simulink model "segway_control"  (R2019b)
settings: Solver=ode45  StartTime=0.0  StopTime=5  MaxStep=0.01  RelTol=1e-3
values from neighbouring files (symbols this model uses):
  A_pitch = [0    1     0     0 ... (first row only)    [vehiculo_autobalanceado_ss.m]
  A_yaw = [0  1 ... (first row only)    [vehiculo_autobalanceado_ss.m]
  B_pitch = [0 ... (first row only)    [vehiculo_autobalanceado_ss.m]
  B_yaw = [0 ... (first row only)    [vehiculo_autobalanceado_ss.m]
  C_pitch = [1 0 0 0 ... (first row only)    [vehiculo_autobalanceado_ss.m]
  C_yaw = [1 0]    [vehiculo_autobalanceado_ss.m]
  D_pitch = zeros(2, 1)    [vehiculo_autobalanceado_ss.m]
  D_yaw = 0    [vehiculo_autobalanceado_ss.m]
libraries: simulink x2
settings Model: Creator=crist  LastModifiedBy=crist

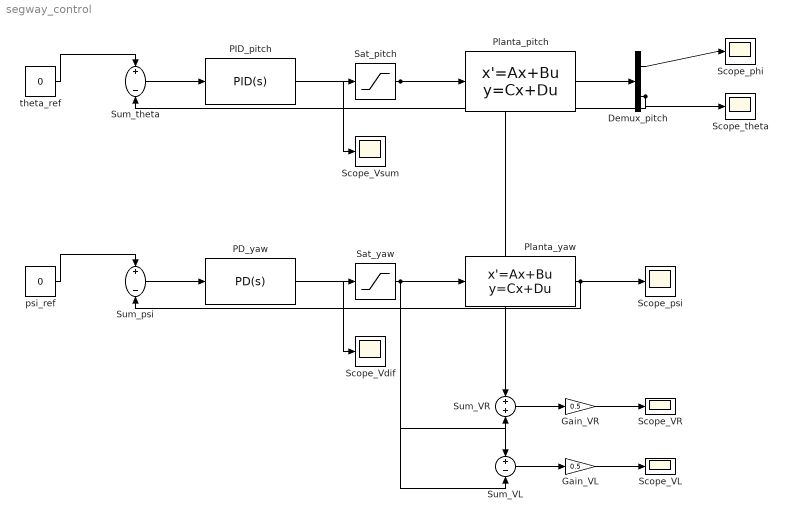
== system segway_control ==
  Demux_pitch : Demux  Outputs=2
  Gain_VL : Gain  Gain=0.5
  Gain_VR : Gain  Gain=0.5
  PD_yaw : simulink/Continuous/PID Controller  Controller=PD  Form=Parallel  TimeDomain=Continuous-time  SampleTime=-1  IntegratorMethod=Forward Euler  FilterMethod=Forward Euler  ControllerParametersSource=internal  P=2  I=1  D=0.3  UseFilter=on  N=100  TunerSelectOption=Transfer Function Based (PID Tuner App)  InitialConditionSource=internal  InitialConditionForIntegrator=0  InitialConditionForFilter=0  DifferentiatorICPrevScaledInput=0  ExternalReset=none  TrackingMode=off  Kt=1  LimitOutput=off  UpperSaturationLimit=inf  LowerSaturationLimit=-inf  LinearizeAsGain=on  AntiWindupMode=none  Kb=1  POutMin=[]  POutMax=[]  IOutMin=[]  IOutMax=[]  DOutMin=[]  DOutMax=[]  NOutMin=[]  NOutMax=[]  SumOutMin=[]  SumOutMax=[]  SaturationOutMin=[]  SaturationOutMax=[]  PParamMin=[]  PParamMax=[]  IParamMin=[]  IParamMax=[]  DParamMin=[]  DParamMax=[]  NParamMin=[]  NParamMax=[]  KbParamMin=[]  KbParamMax=[]  KtParamMin=[]  KtParamMax=[]  KbOutMin=[]  KbOutMax=[]  KtOutMin=[]  KtOutMax=[]  IntegratorOutMin=[]  IntegratorOutMax=[]  FilterOutMin=[]  FilterOutMax=[]  SumI1OutMin=[]  SumI1OutMax=[]  SumI2OutMin=[]  SumI2OutMax=[]  SumI3OutMin=[]  SumI3OutMax=[]  SumI4OutMin=[]  SumI4OutMax=[]  SumDOutMin=[]  SumDOutMax=[]  DifferentiatorOutMin=[]  DifferentiatorOutMax=[]  FilterDiffOutCoefMin=[]  FilterDiffOutCoefMax=[]  ReciprocalOutMin=[]  ReciprocalOutMax=[]  SumDenOutMin=[]  SumDenOutMax=[]  SumNumOutMin=[]  SumNumOutMax=[]  DivideOutMin=[]  DivideOutMax=[]  IntegratorContinuousStateAttributes=''  IntegratorStateMustResolveToSignalObject=off  IntegratorRTWStateStorageClass=Auto  FilterContinuousStateAttributes=''  FilterStateMustResolveToSignalObject=off  FilterRTWStateStorageClass=Auto  ParallelPVariant=InternalParameters  IdealPVariant=Disabled  IVariant=Disabled  DVariant=InternalParameters  IntegratorVariant=Disabled  SatVariant=Disabled  AWVariant=Disabled  PCopyVariant=Disabled  TRVariant=Disabled  FdbkBlocksVariant=Forward  IdealPFdbkVariant=Disabled  SatFdbkVariant=Disabled  DerivativeFilterVariant=ContFilter  NVariant=InternalParameters  NCopyVariant=Disabled  FilterICVariant=InternalICsFilter  IntegratorICVariant=Disabled  ExternalResetVariant=Disabled  TRSumVariant=Passthrough  SumFdbkVariant=Disabled  SumVariant=Sum_PD
  PID_pitch : simulink/Continuous/PID Controller  Controller=PID  Form=Parallel  TimeDomain=Continuous-time  SampleTime=-1  IntegratorMethod=Forward Euler  FilterMethod=Forward Euler  ControllerParametersSource=internal  P=50  I=5  D=8  UseFilter=on  N=100  TunerSelectOption=Transfer Function Based (PID Tuner App)  InitialConditionSource=internal  InitialConditionForIntegrator=0  InitialConditionForFilter=0  DifferentiatorICPrevScaledInput=0  ExternalReset=none  TrackingMode=off  Kt=1  LimitOutput=off  UpperSaturationLimit=inf  LowerSaturationLimit=-inf  LinearizeAsGain=on  AntiWindupMode=none  Kb=1  POutMin=[]  POutMax=[]  IOutMin=[]  IOutMax=[]  DOutMin=[]  DOutMax=[]  NOutMin=[]  NOutMax=[]  SumOutMin=[]  SumOutMax=[]  SaturationOutMin=[]  SaturationOutMax=[]  PParamMin=[]  PParamMax=[]  IParamMin=[]  IParamMax=[]  DParamMin=[]  DParamMax=[]  NParamMin=[]  NParamMax=[]  KbParamMin=[]  KbParamMax=[]  KtParamMin=[]  KtParamMax=[]  KbOutMin=[]  KbOutMax=[]  KtOutMin=[]  KtOutMax=[]  IntegratorOutMin=[]  IntegratorOutMax=[]  FilterOutMin=[]  FilterOutMax=[]  SumI1OutMin=[]  SumI1OutMax=[]  SumI2OutMin=[]  SumI2OutMax=[]  SumI3OutMin=[]  SumI3OutMax=[]  SumI4OutMin=[]  SumI4OutMax=[]  SumDOutMin=[]  SumDOutMax=[]  DifferentiatorOutMin=[]  DifferentiatorOutMax=[]  FilterDiffOutCoefMin=[]  FilterDiffOutCoefMax=[]  ReciprocalOutMin=[]  ReciprocalOutMax=[]  SumDenOutMin=[]  SumDenOutMax=[]  SumNumOutMin=[]  SumNumOutMax=[]  DivideOutMin=[]  DivideOutMax=[]  IntegratorContinuousStateAttributes=''  IntegratorStateMustResolveToSignalObject=off  IntegratorRTWStateStorageClass=Auto  FilterContinuousStateAttributes=''  FilterStateMustResolveToSignalObject=off  FilterRTWStateStorageClass=Auto  ParallelPVariant=InternalParameters  IdealPVariant=Disabled  IVariant=InternalParameters  DVariant=InternalParameters  IntegratorVariant=Continuous  SatVariant=Disabled  AWVariant=Passthrough  PCopyVariant=Disabled  TRVariant=Disabled  FdbkBlocksVariant=Forward  IdealPFdbkVariant=Disabled  SatFdbkVariant=Disabled  DerivativeFilterVariant=ContFilter  NVariant=InternalParameters  NCopyVariant=Disabled  FilterICVariant=InternalICsFilter  IntegratorICVariant=InternalICs  ExternalResetVariant=Disabled  TRSumVariant=Passthrough  SumFdbkVariant=Disabled  SumVariant=Sum_PID
  Planta_pitch : StateSpace  A=A_pitch  B=B_pitch  C=C_pitch  D=D_pitch  InitialCondition=[0; 0; 5*pi/180; 0]
  Planta_yaw : StateSpace  A=A_yaw  B=B_yaw  C=C_yaw  D=D_yaw  InitialCondition=[0; 0]
  Sat_pitch : Saturate  UpperLimit=24  LowerLimit=-24
  Sat_yaw : Saturate  UpperLimit=24  LowerLimit=-24
  Scope_VL : Scope
  Scope_VR : Scope
  Scope_Vdif : Scope
  Scope_Vsum : Scope
  Scope_phi : Scope
  Scope_psi : Scope
  Scope_theta : Scope
  Sum_VL : Sum  Inputs=+-
  Sum_VR : Sum
  Sum_psi : Sum  Inputs=+-
  Sum_theta : Sum  Inputs=+-
  psi_ref : Constant  Value=0
  theta_ref : Constant  Value=0
  wires:
  theta_ref/1 -> Sum_theta/1
  Sum_theta/1 -> PID_pitch/1
  PID_pitch/1 -> Sat_pitch/1
  Sat_pitch/1 -> Planta_pitch/1, Scope_Vsum/1, Sum_VR/1, Sum_VL/1
  Planta_pitch/1 -> Demux_pitch/1
  Demux_pitch/1 -> Scope_phi/1
  Demux_pitch/2 -> Scope_theta/1, Sum_theta/2
  psi_ref/1 -> Sum_psi/1
  Sum_psi/1 -> PD_yaw/1
  PD_yaw/1 -> Sat_yaw/1
  Sat_yaw/1 -> Planta_yaw/1, Scope_Vdif/1, Sum_VR/2, Sum_VL/2
  Planta_yaw/1 -> Scope_psi/1, Sum_psi/2
  Sum_VR/1 -> Gain_VR/1
  Sum_VL/1 -> Gain_VL/1
  Gain_VR/1 -> Scope_VR/1
  Gain_VL/1 -> Scope_VL/1
